simulink model "pi_OfflineRL_H2DF_2023a"  (R2023a)
settings: Solver=FixedStepAuto  StartTime=0.0  StopTime=inf  FixedStep=0.001  RelTol=1e-3  EnableMultiTasking=on
values from neighbouring files (symbols this model uses):
  C2C_NMPC = init_C2C_NMPC_H2DF(C2C_NMPC.expdata)    [init_pi_OfflineRL_H2DF_2023a.m]
  LowerLimit = ([0.17e-3;350;-2;2e-3] - C2C_NMPC.Normalization.controls.mean)./(C2C_NMPC.Normalization.controls.std)    [init_pi_OfflineRL_H2DF_2023a.m]
  UpperLimit = ([0.5e-3;900;10;5.5e-3] - C2C_NMPC.Normalization.controls.mean)./(C2C_NMPC.Normalization.controls.std)    [init_pi_OfflineRL_H2DF_2023a.m]
undefined symbols (not defined in the file or in its folder): DiscIntNeverNeededParam
libraries: deeplib x9, rllib x3, raspberrypiNetworklib x1
(part 4 of 4)

== system pi_OfflineRL_H2DF_2023a/main_C2C/main_C2C_RL/RL_Controller/Subsystem/If Action Subsystem/generate observations ==
  Outputs : Inport
  Reference : Inport  Port=2
  LSTM States : Inport  Port=3
  Abs : Abs  SaturateOnIntegerOverflow=off
  Demux : Demux
  Demux1 : Demux
  Discrete-Time Integrator : DiscreteIntegrator  SampleTime=-1  ICPrevOutput=DiscIntNeverNeededParam  ICPrevScaledInput=DiscIntNeverNeededParam
  Display : Display
  Display1 : Display
  Display2 : Display
  Mux : Mux  Inputs=9
  Selector1 : Selector  IndexOptions=Index vector (dialog)  Indices=[1:4]  OutputSizes=1
  Subtract3 : Sum  Inputs=+-
  Unit Delay : UnitDelay  SampleTime=-1  HasFrameUpgradeWarning=on
  Unit Delay1 : UnitDelay  SampleTime=-1  HasFrameUpgradeWarning=on
  observations : Outport  VectorParamsAs1DForOutWhenUnconnected=off
  wires:
  Mux/1 -> observations/1, Display/1
  Demux1/1 -> Subtract3/2, Mux/1
  Demux1/2 -> Mux/2
  Demux1/3 -> Mux/3
  Demux1/4 -> Mux/4
  Subtract3/1 -> Discrete-Time Integrator/1, Mux/8
  Selector1/1 -> Demux/1, Display1/1
  Demux/1 -> Unit Delay1/1, Mux/6, Unit Delay/1
  Reference/1 -> Selector1/1
  Outputs/1 -> Display2/1, Demux1/1
  Discrete-Time Integrator/1 -> Abs/1
  Unit Delay1/1 -> Subtract3/1
  Unit Delay/1 -> Mux/5
  Abs/1 -> Mux/7
  LSTM States/1 -> Mux/9

== system pi_OfflineRL_H2DF_2023a/main_C2C/main_C2C_RL/post_processing/Subsystem1/Subsystem/ denormalizing reference1 ==
  IMEP_norm : Inport
  NOX_norm : Inport  Port=2
  soot_norm : Inport  Port=3
  MPRR_norm : Inport  Port=4
  Constant : Constant  Value=C2C_NMPC.Normalization.outputs.mean(1)
  Constant1 : Constant  Value=C2C_NMPC.Normalization.outputs.mean(2)
  Constant2 : Constant  Value=C2C_NMPC.Normalization.outputs.mean(3)
  Constant3 : Constant  Value=C2C_NMPC.Normalization.outputs.mean(4)
  Gain : Gain  Gain=C2C_NMPC.Normalization.outputs.std(1)
  Gain1 : Gain  Gain=C2C_NMPC.Normalization.outputs.std(2)
  Gain2 : Gain  Gain=C2C_NMPC.Normalization.outputs.std(3)
  Gain3 : Gain  Gain=C2C_NMPC.Normalization.outputs.std(4)
  Sum{1..3,5} (4 alike) : Sum  Inputs=|++
  IMEP : Outport
  NOX : Outport  Port=2
  soot : Outport  Port=3
  MPRR : Outport  Port=4
  wires:
  Gain/1 -> Sum5/1
  IMEP_norm/1 -> Gain/1
  Constant/1 -> Sum5/2
  Sum5/1 -> IMEP/1
  Gain1/1 -> Sum1/1
  Constant1/1 -> Sum1/2
  NOX_norm/1 -> Gain1/1
  Sum1/1 -> NOX/1
  Gain2/1 -> Sum2/1
  Constant2/1 -> Sum2/2
  soot_norm/1 -> Gain2/1
  Sum2/1 -> soot/1
  Gain3/1 -> Sum3/1
  Constant3/1 -> Sum3/2
  MPRR_norm/1 -> Gain3/1
  Sum3/1 -> MPRR/1

== system pi_OfflineRL_H2DF_2023a/main_C2C/main_C2C_RL/post_processing/Subsystem1/Subsystem/ denormalizing reference2 ==
  IMEP_norm : Inport
  NOX_norm : Inport  Port=2
  soot_norm : Inport  Port=3
  MPRR_norm : Inport  Port=4
  Constant : Constant  Value=C2C_NMPC.Normalization.outputs.mean(1)
  Constant1 : Constant  Value=C2C_NMPC.Normalization.outputs.mean(2)
  Constant2 : Constant  Value=C2C_NMPC.Normalization.outputs.mean(3)
  Constant3 : Constant  Value=C2C_NMPC.Normalization.outputs.mean(4)
  Gain : Gain  Gain=C2C_NMPC.Normalization.outputs.std(1)
  Gain1 : Gain  Gain=C2C_NMPC.Normalization.outputs.std(2)
  Gain2 : Gain  Gain=C2C_NMPC.Normalization.outputs.std(3)
  Gain3 : Gain  Gain=C2C_NMPC.Normalization.outputs.std(4)
  Sum{1..3,5} (4 alike) : Sum  Inputs=|++
  IMEP : Outport
  NOX : Outport  Port=2
  soot : Outport  Port=3
  MPRR : Outport  Port=4
  wires:
  Gain/1 -> Sum5/1
  IMEP_norm/1 -> Gain/1
  Constant/1 -> Sum5/2
  Sum5/1 -> IMEP/1
  Gain1/1 -> Sum1/1
  Constant1/1 -> Sum1/2
  NOX_norm/1 -> Gain1/1
  Sum1/1 -> NOX/1
  Gain2/1 -> Sum2/1
  Constant2/1 -> Sum2/2
  soot_norm/1 -> Gain2/1
  Sum2/1 -> soot/1
  Gain3/1 -> Sum3/1
  Constant3/1 -> Sum3/2
  MPRR_norm/1 -> Gain3/1
  Sum3/1 -> MPRR/1

== system pi_OfflineRL_H2DF_2023a/main_C2C/main_C2C_RL/post_processing/Subsystem1/Subsystem/ denormalizing reference3 ==
  IMEP_norm : Inport
  NOX_norm : Inport  Port=2
  soot_norm : Inport  Port=3
  MPRR_norm : Inport  Port=4
  Constant : Constant  Value=C2C_NMPC.Normalization.outputs.mean(1)
  Constant1 : Constant  Value=C2C_NMPC.Normalization.outputs.mean(2)
  Constant2 : Constant  Value=C2C_NMPC.Normalization.outputs.mean(3)
  Constant3 : Constant  Value=C2C_NMPC.Normalization.outputs.mean(4)
  Gain : Gain  Gain=C2C_NMPC.Normalization.outputs.std(1)
  Gain1 : Gain  Gain=C2C_NMPC.Normalization.outputs.std(2)
  Gain2 : Gain  Gain=C2C_NMPC.Normalization.outputs.std(3)
  Gain3 : Gain  Gain=C2C_NMPC.Normalization.outputs.std(4)
  Sum{1..3,5} (4 alike) : Sum  Inputs=|++
  IMEP : Outport
  NOX : Outport  Port=2
  soot : Outport  Port=3
  MPRR : Outport  Port=4
  wires:
  Gain/1 -> Sum5/1
  IMEP_norm/1 -> Gain/1
  Constant/1 -> Sum5/2
  Sum5/1 -> IMEP/1
  Gain1/1 -> Sum1/1
  Constant1/1 -> Sum1/2
  NOX_norm/1 -> Gain1/1
  Sum1/1 -> NOX/1
  Gain2/1 -> Sum2/1
  Constant2/1 -> Sum2/2
  soot_norm/1 -> Gain2/1
  Sum2/1 -> soot/1
  Gain3/1 -> Sum3/1
  Constant3/1 -> Sum3/2
  MPRR_norm/1 -> Gain3/1
  Sum3/1 -> MPRR/1

== system pi_OfflineRL_H2DF_2023a/main_C2C/main_C2C_RL/post_processing/Subsystem1/Subsystem/ denormalizing reference4 ==
  IMEP_norm : Inport
  NOX_norm : Inport  Port=2
  soot_norm : Inport  Port=3
  MPRR_norm : Inport  Port=4
  Constant : Constant  Value=C2C_NMPC.Normalization.outputs.mean(1)
  Constant1 : Constant  Value=C2C_NMPC.Normalization.outputs.mean(2)
  Constant2 : Constant  Value=C2C_NMPC.Normalization.outputs.mean(3)
  Constant3 : Constant  Value=C2C_NMPC.Normalization.outputs.mean(4)
  Gain : Gain  Gain=C2C_NMPC.Normalization.outputs.std(1)
  Gain1 : Gain  Gain=C2C_NMPC.Normalization.outputs.std(2)
  Gain2 : Gain  Gain=C2C_NMPC.Normalization.outputs.std(3)
  Gain3 : Gain  Gain=C2C_NMPC.Normalization.outputs.std(4)
  Sum{1..3,5} (4 alike) : Sum  Inputs=|++
  IMEP : Outport
  NOX : Outport  Port=2
  soot : Outport  Port=3
  MPRR : Outport  Port=4
  wires:
  Gain/1 -> Sum5/1
  IMEP_norm/1 -> Gain/1
  Constant/1 -> Sum5/2
  Sum5/1 -> IMEP/1
  Gain1/1 -> Sum1/1
  Constant1/1 -> Sum1/2
  NOX_norm/1 -> Gain1/1
  Sum1/1 -> NOX/1
  Gain2/1 -> Sum2/1
  Constant2/1 -> Sum2/2
  soot_norm/1 -> Gain2/1
  Sum2/1 -> soot/1
  Gain3/1 -> Sum3/1
  Constant3/1 -> Sum3/2
  MPRR_norm/1 -> Gain3/1
  Sum3/1 -> MPRR/1

== system pi_OfflineRL_H2DF_2023a/main_C2C_RL/RL_Controller/RL_Controller_ifAction/RL_Controller_PPO1/Subsystem/If Action Subsystem ==
  Reference : Inport
  Outputs : Inport  Port=2
  LSTM States : Inport  Port=3
  Enable : Inport  Port=4
  Action Port : ActionPort  ActionPortLabel=if(u1 > 0)
  generate observations : Subsystem
  observations : Outport
  wires:
  Reference/1 -> generate observations/2(Reference)
  generate observations/1(observations) -> observations/1
  Outputs/1 -> generate observations/1(Outputs)
  Enable/1 -> generate observations/Reset
  LSTM States/1 -> generate observations/3(LSTM States)

== system pi_OfflineRL_H2DF_2023a/main_C2C_RL/RL_Controller/RL_Controller_ifAction/RL_Controller_PPO1/Subsystem/If Action Subsystem1 ==
  Action Port : ActionPort  ActionPortLabel=else
  Constant : Constant  Value=zeros(16,1)
  observations : Outport
  wires:
  Constant/1 -> observations/1

== system pi_OfflineRL_H2DF_2023a/main_C2C_RL/RL_Controller/RL_Controller_ifAction/RL_Controller_PPO2/Subsystem/If Action Subsystem ==
  Reference : Inport
  Outputs : Inport  Port=2
  LSTM States : Inport  Port=3
  Enable : Inport  Port=4
  Action Port : ActionPort  ActionPortLabel=if(u1 > 0)
  generate observations : Subsystem
  observations : Outport
  wires:
  Reference/1 -> generate observations/2(Reference)
  generate observations/1(observations) -> observations/1
  Outputs/1 -> generate observations/1(Outputs)
  Enable/1 -> generate observations/Reset
  LSTM States/1 -> generate observations/3(LSTM States)

== system pi_OfflineRL_H2DF_2023a/main_C2C_RL/RL_Controller/RL_Controller_ifAction/RL_Controller_PPO2/Subsystem/If Action Subsystem1 ==
  Action Port : ActionPort  ActionPortLabel=else
  Constant : Constant  Value=zeros(16,1)
  observations : Outport
  wires:
  Constant/1 -> observations/1

== system pi_OfflineRL_H2DF_2023a/main_C2C_RL/RL_Controller/RL_Controller_ifAction/RL_Controller_PPO3/Subsystem/If Action Subsystem ==
  Reference : Inport
  Outputs : Inport  Port=2
  LSTM States : Inport  Port=3
  Enable : Inport  Port=4
  Action Port : ActionPort  ActionPortLabel=if(u1 > 0)
  generate observations : Subsystem
  observations : Outport
  wires:
  Reference/1 -> generate observations/2(Reference)
  generate observations/1(observations) -> observations/1
  Outputs/1 -> generate observations/1(Outputs)
  Enable/1 -> generate observations/Reset
  LSTM States/1 -> generate observations/3(LSTM States)

== system pi_OfflineRL_H2DF_2023a/main_C2C_RL/RL_Controller/RL_Controller_ifAction/RL_Controller_PPO3/Subsystem/If Action Subsystem1 ==
  Action Port : ActionPort  ActionPortLabel=else
  Constant : Constant  Value=zeros(16,1)
  observations : Outport
  wires:
  Constant/1 -> observations/1

== system pi_OfflineRL_H2DF_2023a/main_C2C_RL/RL_Controller/RL_Controller_ifAction/RL_Controller_PPO4/Subsystem/If Action Subsystem ==
  Reference : Inport
  Outputs : Inport  Port=2
  LSTM States : Inport  Port=3
  Enable : Inport  Port=4
  Action Port : ActionPort  ActionPortLabel=if(u1 > 0)
  generate observations : Subsystem
  observations : Outport
  wires:
  Reference/1 -> generate observations/2(Reference)
  generate observations/1(observations) -> observations/1
  Outputs/1 -> generate observations/1(Outputs)
  Enable/1 -> generate observations/Reset

== system pi_OfflineRL_H2DF_2023a/main_C2C_RL/RL_Controller/RL_Controller_ifAction/RL_Controller_PPO4/Subsystem/If Action Subsystem1 ==
  Action Port : ActionPort  ActionPortLabel=else
  Constant : Constant  Value=zeros(8,1)
  observations : Outport
  wires:
  Constant/1 -> observations/1

== system pi_OfflineRL_H2DF_2023a/main_C2C_RL/RL_Controller/RL_Controller_ifAction/RL_Controller_PPO5/Subsystem/If Action Subsystem ==
  Reference : Inport
  Outputs : Inport  Port=2
  LSTM States : Inport  Port=3
  Enable : Inport  Port=4
  Action Port : ActionPort  ActionPortLabel=if(u1 > 0)
  generate observations : Subsystem
  observations : Outport
  wires:
  Reference/1 -> generate observations/2(Reference)
  generate observations/1(observations) -> observations/1
  Outputs/1 -> generate observations/1(Outputs)
  Enable/1 -> generate observations/Reset

== system pi_OfflineRL_H2DF_2023a/main_C2C_RL/RL_Controller/RL_Controller_ifAction/RL_Controller_PPO5/Subsystem/If Action Subsystem1 ==
  Action Port : ActionPort  ActionPortLabel=else
  Constant : Constant  Value=zeros(8,1)
  observations : Outport
  wires:
  Constant/1 -> observations/1

== system pi_OfflineRL_H2DF_2023a/main_C2C_RL/RL_Controller/RL_Controller_ifAction/RL_Controller_PPO6/Subsystem/If Action Subsystem ==
  Reference : Inport
  Outputs : Inport  Port=2
  LSTM States : Inport  Port=3
  Enable : Inport  Port=4
  Action Port : ActionPort  ActionPortLabel=if(u1 > 0)
  generate observations : Subsystem
  observations : Outport
  wires:
  Reference/1 -> generate observations/2(Reference)
  generate observations/1(observations) -> observations/1
  Outputs/1 -> generate observations/1(Outputs)
  Enable/1 -> generate observations/Reset
  LSTM States/1 -> generate observations/3(LSTM States)

== system pi_OfflineRL_H2DF_2023a/main_C2C_RL/RL_Controller/RL_Controller_ifAction/RL_Controller_PPO6/Subsystem/If Action Subsystem1 ==
  Action Port : ActionPort  ActionPortLabel=else
  Constant : Constant  Value=zeros(16,1)
  observations : Outport
  wires:
  Constant/1 -> observations/1

== system pi_OfflineRL_H2DF_2023a/main_C2C_RL/RL_Controller/RL_Controller_ifAction/RL_Controller_PPO7/Subsystem/If Action Subsystem ==
  Reference : Inport
  Outputs : Inport  Port=2
  LSTM States : Inport  Port=3
  Enable : Inport  Port=4
  Action Port : ActionPort  ActionPortLabel=if(u1 > 0)
  generate observations : Subsystem
  observations : Outport
  wires:
  Reference/1 -> generate observations/2(Reference)
  generate observations/1(observations) -> observations/1
  Outputs/1 -> generate observations/1(Outputs)
  Enable/1 -> generate observations/Reset
  LSTM States/1 -> generate observations/3(LSTM States)

== system pi_OfflineRL_H2DF_2023a/main_C2C_RL/RL_Controller/RL_Controller_ifAction/RL_Controller_PPO7/Subsystem/If Action Subsystem1 ==
  Action Port : ActionPort  ActionPortLabel=else
  Constant : Constant  Value=zeros(16,1)
  observations : Outport
  wires:
  Constant/1 -> observations/1

== system pi_OfflineRL_H2DF_2023a/main_C2C_RL/RL_Controller/RL_Controller_ifAction/RL_Controller_PPO8/Subsystem/If Action Subsystem ==
  Reference : Inport
  Outputs : Inport  Port=2
  LSTM States : Inport  Port=3
  Enable : Inport  Port=4
  Action Port : ActionPort  ActionPortLabel=if(u1 > 0)
  generate observations : Subsystem
  observations : Outport
  wires:
  Reference/1 -> generate observations/2(Reference)
  generate observations/1(observations) -> observations/1
  Outputs/1 -> generate observations/1(Outputs)
  Enable/1 -> generate observations/Reset

== system pi_OfflineRL_H2DF_2023a/main_C2C_RL/RL_Controller/RL_Controller_ifAction/RL_Controller_PPO8/Subsystem/If Action Subsystem1 ==
  Action Port : ActionPort  ActionPortLabel=else
  Constant : Constant  Value=zeros(8,1)
  observations : Outport
  wires:
  Constant/1 -> observations/1

== system pi_OfflineRL_H2DF_2023a/main_C2C_RL/RL_Controller/RL_Controller_ifAction/RL_Controller_PPO1/Subsystem/If Action Subsystem/generate observations ==
  Outputs : Inport
  Reference : Inport  Port=2
  LSTM States : Inport  Port=3
  Reset : ResetPort  DisableCoverage=on
  Demux : Demux
  Demux1 : Demux
  Display : Display
  Display1 : Display
  Display2 : Display
  Mux : Mux  Inputs=9
  Selector1 : Selector  IndexOptions=Index vector (dialog)  Indices=[1:4]  OutputSizes=1
  Subtract1 : Sum  Inputs=+-
  Subtract2 : Sum  Inputs=+-
  Subtract3 : Sum  Inputs=+-
  Unit Delay{,1..3} (4 alike) : UnitDelay  SampleTime=-1  HasFrameUpgradeWarning=on
  observations : Outport  VectorParamsAs1DForOutWhenUnconnected=off
  wires:
  Mux/1 -> observations/1, Display/1
  Demux1/2 -> Unit Delay2/1, Subtract1/2, Mux/2
  Demux1/4 -> Mux/4
  Subtract3/1 -> Mux/8
  Selector1/1 -> Demux/1, Display1/1
  Demux/1 -> Unit Delay1/1, Mux/6, Unit Delay/1
  Reference/1 -> Selector1/1
  Outputs/1 -> Display2/1, Demux1/1
  Unit Delay1/1 -> Subtract3/1
  Unit Delay/1 -> Mux/5
  Subtract2/1 -> Mux/7
  Unit Delay2/1 -> Subtract1/1
  Subtract1/1 -> Mux/3
  Demux1/1 -> Subtract2/1, Unit Delay3/1, Subtract3/2, Mux/1
  Unit Delay3/1 -> Subtract2/2
  LSTM States/1 -> Mux/9

== system pi_OfflineRL_H2DF_2023a/main_C2C_RL/RL_Controller/RL_Controller_ifAction/RL_Controller_PPO2/Subsystem/If Action Subsystem/generate observations ==
  Outputs : Inport
  Reference : Inport  Port=2
  LSTM States : Inport  Port=3
  Reset : ResetPort  DisableCoverage=on
  Demux : Demux
  Demux1 : Demux
  Display : Display
  Display1 : Display
  Display2 : Display
  Mux : Mux  Inputs=9
  Selector1 : Selector  IndexOptions=Index vector (dialog)  Indices=[1:4]  OutputSizes=1
  Subtract1 : Sum  Inputs=+-
  Subtract2 : Sum  Inputs=+-
  Subtract3 : Sum  Inputs=+-
  Unit Delay{,1..3} (4 alike) : UnitDelay  SampleTime=-1  HasFrameUpgradeWarning=on
  observations : Outport  VectorParamsAs1DForOutWhenUnconnected=off
  wires:
  Mux/1 -> observations/1, Display/1
  Demux1/2 -> Unit Delay2/1, Subtract1/2, Mux/2
  Demux1/4 -> Mux/4
  Subtract3/1 -> Mux/8
  Selector1/1 -> Demux/1, Display1/1
  Demux/1 -> Unit Delay1/1, Mux/6, Unit Delay/1
  Reference/1 -> Selector1/1
  Outputs/1 -> Display2/1, Demux1/1
  Unit Delay1/1 -> Subtract3/1
  Unit Delay/1 -> Mux/5
  Subtract2/1 -> Mux/7
  Unit Delay2/1 -> Subtract1/1
  Subtract1/1 -> Mux/3
  Demux1/1 -> Subtract2/1, Unit Delay3/1, Subtract3/2, Mux/1
  Unit Delay3/1 -> Subtract2/2
  LSTM States/1 -> Mux/9

== system pi_OfflineRL_H2DF_2023a/main_C2C_RL/RL_Controller/RL_Controller_ifAction/RL_Controller_PPO3/Subsystem/If Action Subsystem/generate observations ==
  Outputs : Inport
  Reference : Inport  Port=2
  LSTM States : Inport  Port=3
  Reset : ResetPort  DisableCoverage=on
  Demux : Demux
  Demux1 : Demux
  Display : Display
  Display1 : Display
  Display2 : Display
  Mux : Mux  Inputs=9
  Selector1 : Selector  IndexOptions=Index vector (dialog)  Indices=[1:4]  OutputSizes=1
  Subtract1 : Sum  Inputs=+-
  Subtract2 : Sum  Inputs=+-
  Subtract3 : Sum  Inputs=+-
  Unit Delay{,1..3} (4 alike) : UnitDelay  SampleTime=-1  HasFrameUpgradeWarning=on
  observations : Outport  VectorParamsAs1DForOutWhenUnconnected=off
  wires:
  Mux/1 -> observations/1, Display/1
  Demux1/2 -> Unit Delay2/1, Subtract1/2, Mux/2
  Demux1/4 -> Mux/4
  Subtract3/1 -> Mux/8
  Selector1/1 -> Demux/1, Display1/1
  Demux/1 -> Unit Delay1/1, Mux/6, Unit Delay/1
  Reference/1 -> Selector1/1
  Outputs/1 -> Display2/1, Demux1/1
  Unit Delay1/1 -> Subtract3/1
  Unit Delay/1 -> Mux/5
  Subtract2/1 -> Mux/7
  Unit Delay2/1 -> Subtract1/1
  Subtract1/1 -> Mux/3
  Demux1/1 -> Subtract2/1, Unit Delay3/1, Subtract3/2, Mux/1
  Unit Delay3/1 -> Subtract2/2
  LSTM States/1 -> Mux/9

== system pi_OfflineRL_H2DF_2023a/main_C2C_RL/RL_Controller/RL_Controller_ifAction/RL_Controller_PPO4/Subsystem/If Action Subsystem/generate observations ==
  Outputs : Inport
  Reference : Inport  Port=2
  Reset : ResetPort  DisableCoverage=on
  Demux : Demux
  Demux1 : Demux
  Display : Display
  Display1 : Display
  Display2 : Display
  Mux : Mux  Inputs=8
  Selector1 : Selector  IndexOptions=Index vector (dialog)  Indices=[1:4]  OutputSizes=1
  Subtract1 : Sum  Inputs=+-
  Subtract2 : Sum  Inputs=+-
  Subtract3 : Sum  Inputs=+-
  Unit Delay{,1..3} (4 alike) : UnitDelay  SampleTime=-1  HasFrameUpgradeWarning=on
  observations : Outport  VectorParamsAs1DForOutWhenUnconnected=off
  wires:
  Mux/1 -> observations/1, Display/1
  Demux1/2 -> Unit Delay2/1, Subtract1/2, Mux/2
  Demux1/4 -> Mux/4
  Subtract3/1 -> Mux/8
  Selector1/1 -> Demux/1, Display1/1
  Demux/1 -> Unit Delay1/1, Mux/6, Unit Delay/1
  Reference/1 -> Selector1/1
  Outputs/1 -> Display2/1, Demux1/1
  Unit Delay1/1 -> Subtract3/1
  Unit Delay/1 -> Mux/5
  Subtract2/1 -> Mux/7
  Unit Delay2/1 -> Subtract1/1
  Subtract1/1 -> Mux/3
  Demux1/1 -> Subtract2/1, Unit Delay3/1, Subtract3/2, Mux/1
  Unit Delay3/1 -> Subtract2/2

== system pi_OfflineRL_H2DF_2023a/main_C2C_RL/RL_Controller/RL_Controller_ifAction/RL_Controller_PPO5/Subsystem/If Action Subsystem/generate observations ==
  Outputs : Inport
  Reference : Inport  Port=2
  Reset : ResetPort  DisableCoverage=on
  Demux : Demux
  Demux1 : Demux
  Display : Display
  Display1 : Display
  Display2 : Display
  Mux : Mux  Inputs=8
  Selector1 : Selector  IndexOptions=Index vector (dialog)  Indices=[1:4]  OutputSizes=1
  Subtract1 : Sum  Inputs=+-
  Subtract2 : Sum  Inputs=+-
  Subtract3 : Sum  Inputs=+-
  Unit Delay{,1..3} (4 alike) : UnitDelay  SampleTime=-1  HasFrameUpgradeWarning=on
  observations : Outport  VectorParamsAs1DForOutWhenUnconnected=off
  wires:
  Mux/1 -> observations/1, Display/1
  Demux1/2 -> Unit Delay2/1, Subtract1/2, Mux/2
  Demux1/4 -> Mux/4
  Subtract3/1 -> Mux/8
  Selector1/1 -> Demux/1, Display1/1
  Demux/1 -> Unit Delay1/1, Mux/6, Unit Delay/1
  Reference/1 -> Selector1/1
  Outputs/1 -> Display2/1, Demux1/1
  Unit Delay1/1 -> Subtract3/1
  Unit Delay/1 -> Mux/5
  Subtract2/1 -> Mux/7
  Unit Delay2/1 -> Subtract1/1
  Subtract1/1 -> Mux/3
  Demux1/1 -> Subtract2/1, Unit Delay3/1, Subtract3/2, Mux/1
  Unit Delay3/1 -> Subtract2/2

== system pi_OfflineRL_H2DF_2023a/main_C2C_RL/RL_Controller/RL_Controller_ifAction/RL_Controller_PPO6/Subsystem/If Action Subsystem/generate observations ==
  Outputs : Inport
  Reference : Inport  Port=2
  LSTM States : Inport  Port=3
  Reset : ResetPort  DisableCoverage=on
  Demux : Demux
  Demux1 : Demux
  Display : Display
  Display1 : Display
  Display2 : Display
  Mux : Mux  Inputs=9
  Selector1 : Selector  IndexOptions=Index vector (dialog)  Indices=[1:4]  OutputSizes=1
  Subtract1 : Sum  Inputs=+-
  Subtract2 : Sum  Inputs=+-
  Subtract3 : Sum  Inputs=+-
  Unit Delay{,1..3} (4 alike) : UnitDelay  SampleTime=-1  HasFrameUpgradeWarning=on
  observations : Outport  VectorParamsAs1DForOutWhenUnconnected=off
  wires:
  Mux/1 -> observations/1, Display/1
  Demux1/2 -> Unit Delay2/1, Subtract1/2, Mux/2
  Demux1/4 -> Mux/4
  Subtract3/1 -> Mux/8
  Selector1/1 -> Demux/1, Display1/1
  Demux/1 -> Unit Delay1/1, Mux/6, Unit Delay/1
  Reference/1 -> Selector1/1
  Outputs/1 -> Display2/1, Demux1/1
  Unit Delay1/1 -> Subtract3/1
  Unit Delay/1 -> Mux/5
  Subtract2/1 -> Mux/7
  Unit Delay2/1 -> Subtract1/1
  Subtract1/1 -> Mux/3
  Demux1/1 -> Subtract2/1, Unit Delay3/1, Subtract3/2, Mux/1
  Unit Delay3/1 -> Subtract2/2
  LSTM States/1 -> Mux/9

== system pi_OfflineRL_H2DF_2023a/main_C2C_RL/RL_Controller/RL_Controller_ifAction/RL_Controller_PPO7/Subsystem/If Action Subsystem/generate observations ==
  Outputs : Inport
  Reference : Inport  Port=2
  LSTM States : Inport  Port=3
  Reset : ResetPort  DisableCoverage=on
  Demux : Demux
  Demux1 : Demux
  Display : Display
  Display1 : Display
  Display2 : Display
  Mux : Mux  Inputs=9
  Selector1 : Selector  IndexOptions=Index vector (dialog)  Indices=[1:4]  OutputSizes=1
  Subtract1 : Sum  Inputs=+-
  Subtract2 : Sum  Inputs=+-
  Subtract3 : Sum  Inputs=+-
  Unit Delay{,1..3} (4 alike) : UnitDelay  SampleTime=-1  HasFrameUpgradeWarning=on
  observations : Outport  VectorParamsAs1DForOutWhenUnconnected=off
  wires:
  Mux/1 -> observations/1, Display/1
  Demux1/2 -> Unit Delay2/1, Subtract1/2, Mux/2
  Demux1/4 -> Mux/4
  Subtract3/1 -> Mux/8
  Selector1/1 -> Demux/1, Display1/1
  Demux/1 -> Unit Delay1/1, Mux/6, Unit Delay/1
  Reference/1 -> Selector1/1
  Outputs/1 -> Display2/1, Demux1/1
  Unit Delay1/1 -> Subtract3/1
  Unit Delay/1 -> Mux/5
  Subtract2/1 -> Mux/7
  Unit Delay2/1 -> Subtract1/1
  Subtract1/1 -> Mux/3
  Demux1/1 -> Subtract2/1, Unit Delay3/1, Subtract3/2, Mux/1
  Unit Delay3/1 -> Subtract2/2
  LSTM States/1 -> Mux/9

== system pi_OfflineRL_H2DF_2023a/main_C2C_RL/RL_Controller/RL_Controller_ifAction/RL_Controller_PPO8/Subsystem/If Action Subsystem/generate observations ==
  Outputs : Inport
  Reference : Inport  Port=2
  Reset : ResetPort  DisableCoverage=on
  Demux : Demux
  Demux1 : Demux
  Display : Display
  Display1 : Display
  Display2 : Display
  Mux : Mux  Inputs=8
  Selector1 : Selector  IndexOptions=Index vector (dialog)  Indices=[1:4]  OutputSizes=1
  Subtract1 : Sum  Inputs=+-
  Subtract2 : Sum  Inputs=+-
  Subtract3 : Sum  Inputs=+-
  Unit Delay{,1..3} (4 alike) : UnitDelay  SampleTime=-1  HasFrameUpgradeWarning=on
  observations : Outport  VectorParamsAs1DForOutWhenUnconnected=off
  wires:
  Mux/1 -> observations/1, Display/1
  Demux1/2 -> Unit Delay2/1, Subtract1/2, Mux/2
  Demux1/4 -> Mux/4
  Subtract3/1 -> Mux/8
  Selector1/1 -> Demux/1, Display1/1
  Demux/1 -> Unit Delay1/1, Mux/6, Unit Delay/1
  Reference/1 -> Selector1/1
  Outputs/1 -> Display2/1, Demux1/1
  Unit Delay1/1 -> Subtract3/1
  Unit Delay/1 -> Mux/5
  Subtract2/1 -> Mux/7
  Unit Delay2/1 -> Subtract1/1
  Subtract1/1 -> Mux/3
  Demux1/1 -> Subtract2/1, Unit Delay3/1, Subtract3/2, Mux/1
  Unit Delay3/1 -> Subtract2/2

== stateflow chart pi_OfflineRL_H2DF_2023a/Chart1 ==
  state wait
  (default) -> wait
  wait -> (junction 9) : [size>0]{call_main_C2C; call_tx_C2C}
  (junction 10) -> wait
  (junction 9) -> (junction 10)
  data: size input
  events: call_tx_C2C output FUNCTION_CALL_EVENT; call_main_C2C output FUNCTION_CALL_EVENT

== matlab function pi_OfflineRL_H2DF_2023a/main_C2C_RL/RL_Controller/dyn_H2DF_state_augmentation/dyn_H2DF_state_augmentation ==
  data: last_LSTM_states input; LSTM_states output; controls input; last_outputs input; H2DF_Par parameter
function LSTM_states = dyn_H2DF_state_augmentation(last_LSTM_states, controls, last_outputs, H2DF_Par)

LSTM_states = dyn_H2DF_state_augmentation_GRU(last_LSTM_states,[controls; last_outputs(1)], H2DF_Par);

== matlab function pi_OfflineRL_H2DF_2023a/main_C2C_RL/RL_Controller/State_Augmentation/dyn_H2DF/dyn_H2DF ==
  data: last_LSTM_states input; controls input; outputs output; last_outputs input; H2DF_Par parameter; LSTM_states output
 function [outputs, LSTM_states] = dyn_H2DF(last_LSTM_states, controls, last_outputs, H2DF_Par)

[outputs, LSTM_states] = dyn_H2DF_GRU(last_LSTM_states, [controls; last_outputs(1)], H2DF_Par);

== matlab function pi_OfflineRL_H2DF_2023a/main_C2C_RL/RL_Controller/State_Augmentation/dyn_H2DF_state_augmentation/dyn_H2DF_state_augmentation ==
  data: last_LSTM_states input; LSTM_states output; controls input; last_outputs input; H2DF_Par parameter
function LSTM_states = dyn_H2DF_state_augmentation(last_LSTM_states, controls, last_outputs, H2DF_Par)

LSTM_states = dyn_H2DF_state_augmentation_GRU(last_LSTM_states,[controls; last_outputs(1)], H2DF_Par);

== matlab function pi_OfflineRL_H2DF_2023a/tx_C2C/tx_C2C_n3/encode ==
  data: data input; serialized_data output
function serialized_data = encode_to_udp_send(data)

% data is sent as 4 byte (32 bit) packets (uint32)
% 8 byte (64 bit) per double -> 2 packets per double
n_32_bit_packets_per_double = 2;

n_doubles = length(data);
n_32_bit_packets = n_doubles * n_32_bit_packets_per_double;

serialized_data = uint32(zeros(n_32_bit_packets, 1));
for idx = 1:n_doubles
    packet_indices = (idx - 1) * n_32_bit_packets_per_double + 1:(idx * n_32_bit_packets_per_double);
    serialized_data(packet_indices) = typecast(data(idx), 'uint32');
end

== matlab function pi_OfflineRL_H2DF_2023a/main_C2C/main_C2C_RL/RL_Controller/State_Augmentation/dyn_H2DF/dyn_H2DF ==
  data: last_LSTM_states input; controls input; outputs output; last_outputs input; H2DF_Par parameter; LSTM_states output
 function [outputs, LSTM_states] = dyn_H2DF(last_LSTM_states, controls, last_outputs, H2DF_Par)

[outputs, LSTM_states] = dyn_H2DF_GRU(last_LSTM_states, [controls; last_outputs(1)], H2DF_Par);

== matlab function pi_OfflineRL_H2DF_2023a/main_C2C/main_C2C_RL/RL_Controller/State_Augmentation/dyn_H2DF_state_augmentation/dyn_H2DF_state_augmentation ==
  data: last_LSTM_states input; LSTM_states output; controls input; last_outputs input; H2DF_Par parameter
function LSTM_states = dyn_H2DF_state_augmentation(last_LSTM_states, controls, last_outputs, H2DF_Par)

LSTM_states = dyn_H2DF_state_augmentation_GRU(last_LSTM_states,[controls; last_outputs(1)], H2DF_Par);

== matlab function pi_OfflineRL_H2DF_2023a/tx_C2C/tx_C2C_n3_GRU/encode ==
  data: data input; serialized_data output
function serialized_data = encode_to_udp_send(data)

% data is sent as 4 byte (32 bit) packets (uint32)
% 8 byte (64 bit) per double -> 2 packets per double
n_32_bit_packets_per_double = 2;

n_doubles = length(data);
n_32_bit_packets = n_doubles * n_32_bit_packets_per_double;

serialized_data = uint32(zeros(n_32_bit_packets, 1));
for idx = 1:n_doubles
    packet_indices = (idx - 1) * n_32_bit_packets_per_double + 1:(idx * n_32_bit_packets_per_double);
    serialized_data(packet_indices) = typecast(data(idx), 'uint32');
end
